simulink model "Directcurrentcontrol_STATCOM1_PF_send"  (Simulink 8.5)
settings: Solver=ode3  StartTime=0.0  StopTime=0.2  FixedStep=20e-6  RelTol=1e-3
undefined symbols (not defined in the file): D1, Delta
libraries: powerlib x36, powerlib_extras x8, powerlib_meascontrol x5, simulink x3
settings Model: Creator=User  LastModifiedBy=DELL
settings DebuggingCC: SolverPrmCheckMsg=warning  FcnCallInpInsideContextMsg=EnableAllAsWarning

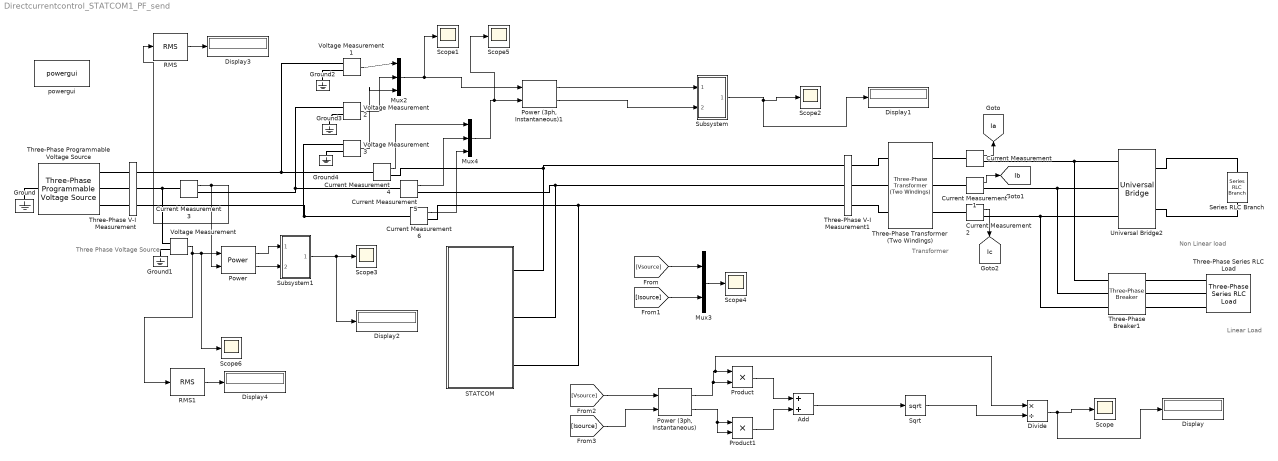
== system Directcurrentcontrol_STATCOM1_PF_send ==
  note: Transformer
  note: Non Linear load
  note: Linear Load
  note: Three Phase Voltage Source
  Add : Sum
  Current Measurement{,1..6} (7 alike) : powerlib/Measurements/Current Measurement  PhasorSimulation=off  OutputType=Complex  PSBequivalent=0
  Display{,1..4} (5 alike) : Display
  Divide : Product  Inputs=*/
  Ground{,1..4} (5 alike) : powerlib/Elements/Ground  LConnTagsString=a
  Mux2 : Mux  Inputs=3
  Mux3 : Mux  Inputs=2
  Mux4 : Mux  Inputs=3
  Power : powerlib_meascontrol/Measurements/Power  Freq=60  Vinit=[1, 0]  Iinit=[1, 0]  Ts=0
  "Power (3ph, Instantaneous)" : powerlib_meascontrol/Measurements/Power (3ph, Instantaneous)
  "Power (3ph, Instantaneous)1" : powerlib_meascontrol/Measurements/Power (3ph, Instantaneous)
  Product : Product
  Product1 : Product
  RMS : powerlib_meascontrol/Measurements/RMS  TrueRMS=on  Freq=60  RMSInit=120  Ts=0
  RMS1 : powerlib_meascontrol/Measurements/RMS  TrueRMS=on  Freq=60  RMSInit=120  Ts=0
  STATCOM : Subsystem
  Scope{,1..6} (7 alike) : Scope
      Scope settings: SaveName=ScopeData4
      Scope1 settings: TimeRange=0.1  YMin=0.86  YMax=1  SaveName=ScopeData2
      Scope2 settings: TimeRange=0.1  YMin=0.86  YMax=1  SaveName=ScopeData6
      Scope3 settings: TimeRange=0.1  YMin=0.86  YMax=1  SaveName=ScopeData11
      Scope4 settings: YMin=-126.5  YMax=-121.5  SaveName=ScopeData7
      Scope5 settings: TimeRange=0.1  YMin=0.86  YMax=1  SaveName=ScopeData12
      Scope6 settings: TimeRange=0.1  YMin=0.86  YMax=1  SaveName=ScopeData13
  Series RLC Branch : powerlib/Elements/Series RLC Branch  LConnTagsString=__new0  RConnTagsString=__new0  BranchType=RL  Resistance=15  Inductance=100e-3  SetiL0=off  InitialCurrent=0  Capacitance=1e-6  Setx0=off  InitialVoltage=0  Measurements=None
  Sqrt : Sqrt  SaturateOnIntegerOverflow=on
  Subsystem : Subsystem
  Subsystem1 : Subsystem
  Three-Phase Programmable Voltage Source : powerlib/Electrical Sources/Three-Phase Programmable Voltage Source  PositiveSequence=[440 0 50]  VariationEntity=None  VariationType=Step  VariationTypeAlt=Step  VariationStep=0.5  VariationRate=10  VariationMagnitude=0.3  VariationFrequency=2  VariationTiming=[1 2]  VariationPhaseA=off  Amplitudes=[1 0.8 1.2 1.0]  TimeValues=[0 0.1 0.15 0.2]  HarmonicGeneration=off  HarmonicA=[3 0.2 -25 0]  HarmonicB=[2 0.15 35 2]  Timing="[0.05  3]"  BusType=swing  Pref=0  Qref=0  Qmin=-inf  Qmax=inf
  Three-Phase Series RLC Load : powerlib/Elements/Three-Phase Series RLC Load  LConnTagsString=A|B|C  Configuration=Y (grounded)  NominalVoltage=220  NominalFrequency=50  ActivePower=2e3  InductivePower=5e3  CapacitivePower=0  Measurements=None  LoadType=constant Z
  Three-Phase Transformer (Two Windings) : powerlib/Elements/Three-Phase Transformer (Two Windings)  Winding1Connection=Delta (D1)  Winding2Connection=Delta (D1)  CoreType=Three single-phase transformers  SetSaturation=off  Hysteresis=off  DataFile='hysteresis'  SetInitialFlux=off  Measurements=None  UNITS=pu  NominalPower=[ 10e3 , 50 ]  Winding1=[ 220 , 0.002 , 0.08 ]  Winding2=[ 220 , 0.002 , 0.08 ]  Rm=500  Lm=500  L0=0.5  Saturation=[ 0,0 ; 0.0024,1.2 ; 1.0,1.52 ]  InitialFluxes=[ 0.8 , -0.8 , 0.7 ]  MoreParameters=off  BreakLoop=off  DataType=off  TransfoNumber=1
  Three-Phase V-I Measurement : powerlib/Measurements/Three-Phase V-I Measurement  VoltageMeasurement=phase-to-phase  SetLabelV=on  LabelV=Vsource  Vpu=off  VpuLL=off  CurrentMeasurement=yes  SetLabelI=on  LabelI=Isource  Ipu=off  Pbase=100e6  Vbase=500e3  OutputType=Complex  PhasorSimulation=off  PSBequivalent=0
  Three-Phase V-I Measurement1 : powerlib/Measurements/Three-Phase V-I Measurement  VoltageMeasurement=phase-to-ground  SetLabelV=on  LabelV=Vabc  Vpu=off  VpuLL=off  CurrentMeasurement=yes  SetLabelI=on  LabelI=Iabc  Ipu=off  Pbase=100e6  Vbase=500e3  OutputType=Complex  PhasorSimulation=off  PSBequivalent=0
  Three-Phase Breaker1 : powerlib/Elements/Three-Phase Breaker  InitialState=open  SwitchA=on  SwitchB=on  SwitchC=on  SwitchTimes=0.1  External=off  BreakerResistance=0.001  SnubberResistance=1e6  SnubberCapacitance=inf  Measurements=None
  Universal Bridge2 : powerlib/Power Electronics/Universal Bridge  Arms=3  SnubberResistance=1e5  SnubberCapacitance=inf  Device=Diodes  Ron=1e-3  Lon=0  ForwardVoltages="[  0  0  ]"  ForwardVoltage=0  GTOparameters=[ 10e-6 , 20e-6 ]  IGBTparameters=[ 1e-6 , 2e-6 ]  Measurements=None  Measurements_2=None  converterType=Rectifier
  Voltage Measurement{,1..3} (4 alike) : powerlib/Measurements/Voltage Measurement  PhasorSimulation=off  OutputType=Complex  PSBequivalent=0
  powergui : powerlib/powergui  SimulationMode=Discrete  SolverType=Tustin/Backward Euler (TBE)  SampleTime=20e-6  frequency=60  SPID=off  DisableSnubberDevices=off  DisableRonSwitches=off  DisableVfSwitches=off  SwTol=0  DisplayEquations=off  Interpol=off  methode=off  Ts=0  FunctionMessages=off  echomessages=off  HookPort=off  EnableUseOfTLC=off  x0status=blocks  frequencyindice=0  Pbase=100e6  ErrMax=1e-4  Iterations=50  UnitsV=kV  UnitsW=MW  buscounter=0  RestoreLinks=warning  ResistiveCurrentMeasurement=off  Frange=[0:2:500]  Ylog=off  Xlog=on  ShowGrid=off  save=off  variable=ZData  structure=ScopeData7  ZoomFFT=off  StartTime=0.02  cycles=1  DisplayStyle=1  fundamental=50  FreqAxis=off  MaxFrequency=1000  frequencyindicesteady=1  RmsSteady=1  display=off
  tag scope: Ia=global, Ib=global, Ic=global
  wires:
  Current Measurement/1 -> [Ia]
  Current Measurement1/1 -> [Ib]
  [Vsource] -> Mux3/1
  [Isource] -> Mux3/2
  Mux3/1 -> Scope4/1
  Current Measurement2/1 -> [Ic]
  "Power (3ph, Instantaneous)"/1 -> Divide/1, Product/1, Product/2
  "Power (3ph, Instantaneous)"/2 -> Product1/1, Product1/2
  Product/1 -> Add/1
  Product1/1 -> Add/2
  Add/1 -> Sqrt/1
  Sqrt/1 -> Divide/2
  Divide/1 -> Display/1, Scope/1
  [Vsource] -> "Power (3ph, Instantaneous)"/1
  [Isource] -> "Power (3ph, Instantaneous)"/2
  Voltage Measurement1/1 -> Mux2/1
  Voltage Measurement2/1 -> Mux2/2
  Voltage Measurement3/1 -> Mux2/3
  Current Measurement4/1 -> Mux4/1
  Current Measurement5/1 -> Mux4/2
  Current Measurement6/1 -> Mux4/3
  Mux2/1 -> Scope1/1, "Power (3ph, Instantaneous)1"/1
  Mux4/1 -> Scope5/1, "Power (3ph, Instantaneous)1"/2
  Subsystem/1(Out1) -> Display1/1, Scope2/1
  "Power (3ph, Instantaneous)1"/1 -> Subsystem/1(In1)
  "Power (3ph, Instantaneous)1"/2 -> Subsystem/2(In2)
  Voltage Measurement/1 -> RMS1/1, Scope6/1, Power/1
  Power/1 -> Subsystem1/1(In1)
  Power/2 -> Subsystem1/2(In2)
  Subsystem1/1(Out1) -> Display2/1, Scope3/1
  RMS/1 -> Display3/1
  RMS1/1 -> Display4/1
  Current Measurement3/1 -> Power/2, RMS/1
  connections:
  Current Measurement6/RConn1 -- STATCOM/RConn3 -- Three-Phase V-I Measurement1/LConn3
  Current Measurement5/RConn1 -- STATCOM/RConn2 -- Three-Phase V-I Measurement1/LConn2
  Universal Bridge2/LConn2 -- Current Measurement1/RConn1 -- Three-Phase Breaker1/LConn2
  Current Measurement/RConn1 -- Universal Bridge2/LConn1 -- Three-Phase Breaker1/LConn1
  Three-Phase Programmable Voltage Source/RConn1 -- Three-Phase V-I Measurement/LConn1
  Three-Phase Programmable Voltage Source/RConn2 -- Three-Phase V-I Measurement/LConn2
  Three-Phase Programmable Voltage Source/RConn3 -- Three-Phase V-I Measurement/LConn3
  Three-Phase V-I Measurement1/RConn1 -- Three-Phase Transformer (Two Windings)/LConn1
  Three-Phase V-I Measurement1/RConn2 -- Three-Phase Transformer (Two Windings)/LConn2
  Three-Phase V-I Measurement1/RConn3 -- Three-Phase Transformer (Two Windings)/LConn3
  Three-Phase Breaker1/RConn1 -- Three-Phase Series RLC Load/LConn1
  Three-Phase Breaker1/RConn2 -- Three-Phase Series RLC Load/LConn2
  Three-Phase Breaker1/RConn3 -- Three-Phase Series RLC Load/LConn3
  Ground/LConn1 -- Three-Phase Programmable Voltage Source/LConn1
  Three-Phase Transformer (Two Windings)/RConn2 -- Current Measurement1/LConn1
  Three-Phase Transformer (Two Windings)/RConn3 -- Current Measurement2/LConn1
  Universal Bridge2/RConn1 -- Series RLC Branch/LConn1
  Current Measurement/LConn1 -- Three-Phase Transformer (Two Windings)/RConn1
  Universal Bridge2/RConn2 -- Series RLC Branch/RConn1
  Current Measurement2/RConn1 -- Universal Bridge2/LConn3 -- Three-Phase Breaker1/LConn3
  Voltage Measurement1/LConn1 -- Three-Phase V-I Measurement/RConn1 -- Current Measurement4/LConn1
  Voltage Measurement/LConn2 -- Ground1/LConn1
  Ground2/LConn1 -- Voltage Measurement1/LConn2
  Voltage Measurement2/LConn2 -- Ground3/LConn1
  Voltage Measurement3/LConn2 -- Ground4/LConn1
  Current Measurement4/RConn1 -- Three-Phase V-I Measurement1/LConn1 -- STATCOM/RConn1
  Voltage Measurement3/LConn1 -- Three-Phase V-I Measurement/RConn3 -- Current Measurement6/LConn1
  Voltage Measurement2/LConn1 -- Current Measurement3/RConn1 -- Current Measurement5/LConn1
  Current Measurement3/LConn1 -- Three-Phase V-I Measurement/RConn2 -- Voltage Measurement/LConn1

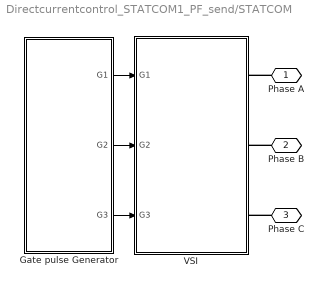
== system Directcurrentcontrol_STATCOM1_PF_send/STATCOM ==
  Gate pulse Generator : Subsystem
  VSI : Subsystem
  Phase A : PMIOPort  Port=1  Side=Right
  Phase B : PMIOPort  Port=2  Side=Right
  Phase C : PMIOPort  Port=3  Side=Right
  wires:
  Gate pulse Generator/1(G1) -> VSI/1(G1)
  Gate pulse Generator/2(G2) -> VSI/2(G2)
  Gate pulse Generator/3(G3) -> VSI/3(G3)
  connections:
  Phase A/RConn1 -- VSI/RConn1
  Phase B/RConn1 -- VSI/RConn2
  Phase C/RConn1 -- VSI/RConn3

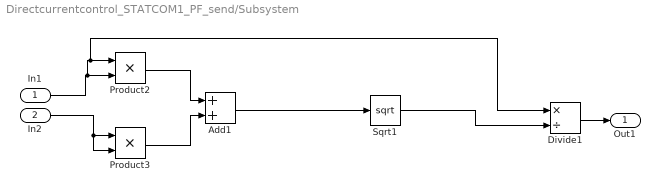
== system Directcurrentcontrol_STATCOM1_PF_send/Subsystem ==
  In1 : Inport
  In2 : Inport  Port=2
  Add1 : Sum
  Divide1 : Product  Inputs=*/
  Product2 : Product
  Product3 : Product
  Sqrt1 : Sqrt  SaturateOnIntegerOverflow=on
  Out1 : Outport
  wires:
  Sqrt1/1 -> Divide1/2
  Product2/1 -> Add1/1
  Product3/1 -> Add1/2
  Add1/1 -> Sqrt1/1
  In1/1 -> Divide1/1, Product2/1, Product2/2
  Divide1/1 -> Out1/1
  In2/1 -> Product3/1, Product3/2

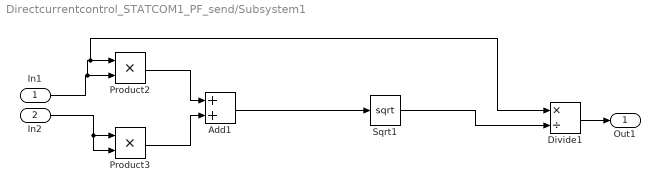
== system Directcurrentcontrol_STATCOM1_PF_send/Subsystem1 ==
  In1 : Inport
  In2 : Inport  Port=2
  Add1 : Sum
  Divide1 : Product  Inputs=*/
  Product2 : Product
  Product3 : Product
  Sqrt1 : Sqrt  SaturateOnIntegerOverflow=on
  Out1 : Outport
  wires:
  Sqrt1/1 -> Divide1/2
  Product2/1 -> Add1/1
  Product3/1 -> Add1/2
  Add1/1 -> Sqrt1/1
  In1/1 -> Divide1/1, Product2/1, Product2/2
  Divide1/1 -> Out1/1
  In2/1 -> Product3/1, Product3/2

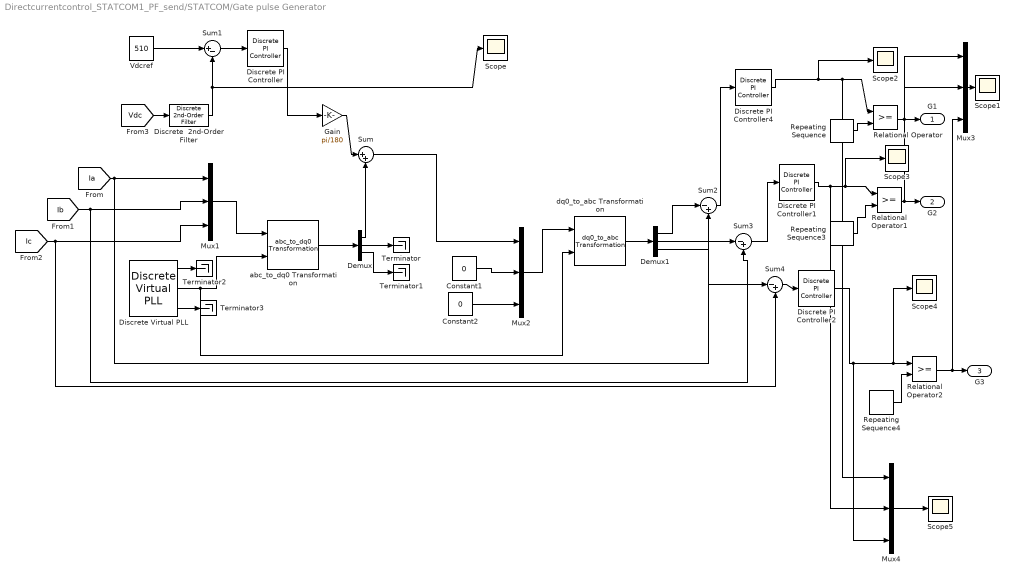
== system Directcurrentcontrol_STATCOM1_PF_send/STATCOM/Gate pulse Generator ==
  Constant1 : Constant  Value=0
  Constant2 : Constant  Value=0
  Demux : Demux  Outputs=3
  Demux1 : Demux  Outputs=3
  Discrete PI Controller : powerlib_extras/Discrete  Control Blocks/Discrete PI Controller  Kp=0.1  Ki=0.005  Par_Limits=[1 -1]  Init=0  Ts=20e-6
  Discrete PI Controller1 : powerlib_extras/Discrete  Control Blocks/Discrete PI Controller  Kp=0.05  Ki=0.05  Par_Limits=[1 -1]  Init=0  Ts=20e-6
  Discrete PI Controller2 : powerlib_extras/Discrete  Control Blocks/Discrete PI Controller  Kp=0.05  Ki=0.05  Par_Limits=[1 -1]  Init=0  Ts=20e-6
  Discrete PI Controller4 : powerlib_extras/Discrete  Control Blocks/Discrete PI Controller  Kp=0.05  Ki=0.05  Par_Limits=[1 -1]  Init=0  Ts=20e-6
  Discrete Virtual PLL : powerlib_extras/Discrete  Control Blocks/Discrete Virtual PLL  Freq=50  Phase=0  Ts=20e-6
  Discrete  2nd-Order Filter : powerlib_extras/Discrete  Control Blocks/Discrete  2nd-Order Filter  FilterType=Lowpass  Fo=200  Zeta=0.707  Ts=20e-6  Initialize=off  Vac_Init=[0.8 -25 60]  Vdc_Init=-0.4  PlotResponse=off  param1=[1 500 1]
  Gain : Gain  Gain=pi/180
  Mux{1..4} (4 alike) : Mux  Inputs=3
  Relational Operator : RelationalOperator  OutDataTypeStr='double'
  Relational Operator1 : RelationalOperator  OutDataTypeStr='double'
  Relational Operator2 : RelationalOperator  OutDataTypeStr='double'
  Repeating Sequence : simulink/Sources/Repeating Sequence  rep_seq_t=[0 0.125 0.25]*1e-3  rep_seq_y=[-1 1 -1]
  Repeating Sequence3 : simulink/Sources/Repeating Sequence  rep_seq_t=[0 0.125 0.25]*1e-3  rep_seq_y=[-1 1 -1]
  Repeating Sequence4 : simulink/Sources/Repeating Sequence  rep_seq_t=[0 0.125 0.25]*1e-3  rep_seq_y=[-1 1 -1]
  Scope{,1..5} (6 alike) : Scope
      Scope settings: SaveName=ScopeData5
      Scope2 settings: SaveName=ScopeData8
      Scope3 settings: SaveName=ScopeData9
      Scope4 settings: SaveName=ScopeData10
      Scope5 settings: SaveName=ScopeData3
  Sum : Sum  Inputs=|++
  Sum1 : Sum  Inputs=|+-
  Sum2 : Sum  Inputs=|-+
  Sum3 : Sum  Inputs=|-+
  Sum4 : Sum  Inputs=|-+
  Terminator{,1..3} (4 alike) : Terminator
  Vdcref : Constant  Value=510
  abc_to_dq0 Transformation : powerlib_extras/Measurements/abc_to_dq0 Transformation
  dq0_to_abc Transformation : powerlib_extras/Measurements/dq0_to_abc Transformation
  G1 : Outport
  G2 : Outport  Port=2
  G3 : Outport  Port=3
  wires:
  Discrete Virtual PLL/2 -> abc_to_dq0 Transformation/2, dq0_to_abc Transformation/2
  Mux1/1 -> abc_to_dq0 Transformation/1
  [Ia] -> Mux1/1, Sum2/2
  [Ib] -> Mux1/2, Sum3/2
  [Ic] -> Mux1/3, Sum4/2
  abc_to_dq0 Transformation/1 -> Demux/1
  Sum1/1 -> Discrete PI Controller/1
  Discrete PI Controller/1 -> Gain/1
  Demux/1 -> Sum/2
  Mux2/1 -> dq0_to_abc Transformation/1
  Vdcref/1 -> Sum1/1
  [Vdc] -> Discrete  2nd-Order Filter/1
  Sum/1 -> Mux2/1
  dq0_to_abc Transformation/1 -> Demux1/1
  Demux1/1 -> Sum2/1
  Demux1/2 -> Sum3/1
  Demux1/3 -> Sum4/1
  Repeating Sequence/1 -> Relational Operator/2
  Relational Operator/1 -> G1/1, Mux3/1
  Relational Operator1/1 -> G2/1, Mux3/2
  Relational Operator2/1 -> G3/1, Mux3/3
  Demux/2 -> Terminator/1
  Demux/3 -> Terminator1/1
  Discrete Virtual PLL/1 -> Terminator2/1
  Discrete Virtual PLL/3 -> Terminator3/1
  Constant1/1 -> Mux2/2
  Constant2/1 -> Mux2/3
  Repeating Sequence3/1 -> Relational Operator1/2
  Repeating Sequence4/1 -> Relational Operator2/2
  Sum2/1 -> Discrete PI Controller4/1
  Sum4/1 -> Discrete PI Controller2/1
  Discrete PI Controller1/1 -> Relational Operator1/1, Scope3/1, Mux4/2
  Discrete  2nd-Order Filter/1 -> Sum1/2, Scope/1
  Gain/1 -> Sum/1
  Mux3/1 -> Scope1/1
  Mux4/1 -> Scope5/1
  Discrete PI Controller4/1 -> Scope2/1, Relational Operator/1, Mux4/1
  Sum3/1 -> Discrete PI Controller1/1
  Discrete PI Controller2/1 -> Relational Operator2/1, Scope4/1, Mux4/3

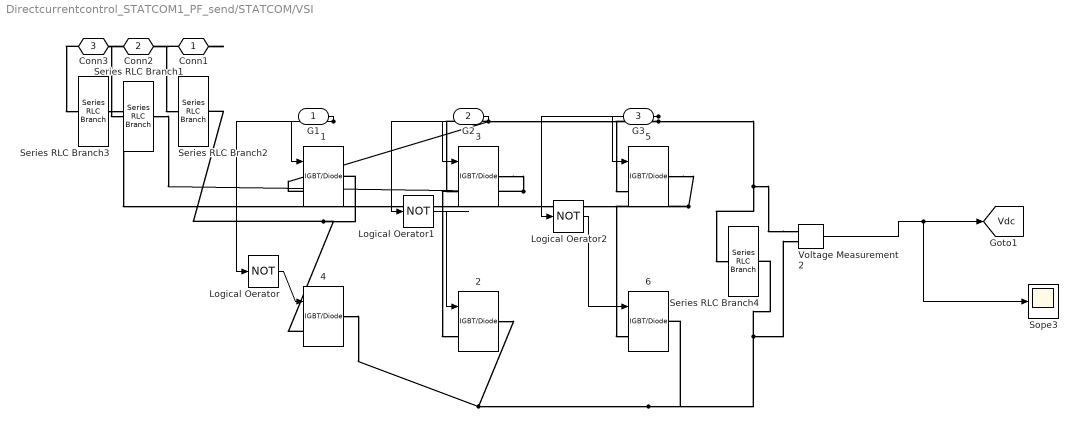
== system Directcurrentcontrol_STATCOM1_PF_send/STATCOM/VSI ==
  G1 : Inport
  G2 : Inport  Port=2
  G3 : Inport  Port=3
  {1..6} (6 alike) : powerlib/Power Electronics/IGBT//Diode  Ron=1e-3  Rs=1e5  Cs=inf  Measurements=off
  Logical Oerator : Logic  Operator=NOT  AllPortsSameDT=off  OutDataTypeStr=boolean
  Logical Oerator1 : Logic  Operator=NOT  AllPortsSameDT=off  OutDataTypeStr=boolean
  Logical Oerator2 : Logic  Operator=NOT  AllPortsSameDT=off  OutDataTypeStr=boolean
  Series RLC Branch1 : powerlib/Elements/Series RLC Branch  LConnTagsString=__new0  RConnTagsString=__new0  BranchType=RL  Resistance=10  Inductance=3e-3  SetiL0=off  InitialCurrent=0  Capacitance=1e-6  Setx0=off  InitialVoltage=0  Measurements=None
  Series RLC Branch2 : powerlib/Elements/Series RLC Branch  LConnTagsString=__new0  RConnTagsString=__new0  BranchType=RL  Resistance=10  Inductance=3e-3  SetiL0=off  InitialCurrent=0  Capacitance=1e-6  Setx0=off  InitialVoltage=0  Measurements=None
  Series RLC Branch3 : powerlib/Elements/Series RLC Branch  LConnTagsString=__new0  RConnTagsString=__new0  BranchType=RL  Resistance=10  Inductance=3e-3  SetiL0=off  InitialCurrent=0  Capacitance=1e-6  Setx0=off  InitialVoltage=0  Measurements=None
  Series RLC Branch4 : powerlib/Elements/Series RLC Branch  LConnTagsString=__new0  RConnTagsString=__new0  BranchType=C  Resistance=1  Inductance=1e-3  SetiL0=off  InitialCurrent=0  Capacitance=2000e-6  Setx0=on  InitialVoltage=500  Measurements=None
  Sope3 : Scope
      settings: YMin=-25  YMax=375
  Voltage Measurement2 : powerlib/Measurements/Voltage Measurement  PhasorSimulation=off  OutputType=Complex  PSBequivalent=0
  Conn1 : PMIOPort  Port=1  Side=Right
  Conn2 : PMIOPort  Port=2  Side=Right
  Conn3 : PMIOPort  Port=3  Side=Right
  tag scope: Vdc=global
  wires:
  G1/1 -> 1/1, Logical Oerator/1
  G2/1 -> 3/1, Logical Oerator1/1
  G3/1 -> 5/1, Logical Oerator2/1
  Logical Oerator/1 -> 4/1
  Logical Oerator1/1 -> 2/1
  Logical Oerator2/1 -> 6/1
  Voltage Measurement2/1 -> [Vdc], Sope3/1
  connections:
  Voltage Measurement2/LConn1 -- 1/LConn1 -- 3/LConn1 -- 5/LConn1 -- Series RLC Branch4/LConn1
  Series RLC Branch2/RConn1 -- 4/LConn1 -- 1/RConn1
  Series RLC Branch1/RConn1 -- 3/RConn1 -- 2/LConn1
  Voltage Measurement2/LConn2 -- Series RLC Branch4/RConn1 -- 4/RConn1 -- 2/RConn1 -- 6/RConn1
  Series RLC Branch3/RConn1 -- 5/RConn1 -- 6/LConn1
  Conn1/RConn1 -- Series RLC Branch2/LConn1
  Conn2/RConn1 -- Series RLC Branch1/LConn1
  Conn3/RConn1 -- Series RLC Branch3/LConn1
